simulink model "Fluxo_de_massa"  (R2025b)
settings: Solver=VariableStepAuto  StartTime=0.0  StopTime=10.0  RelTol=1e-3
undefined symbols (not defined in the file): N, Vd
settings Model: Creator=ivomu  LastModifiedBy=ivomu

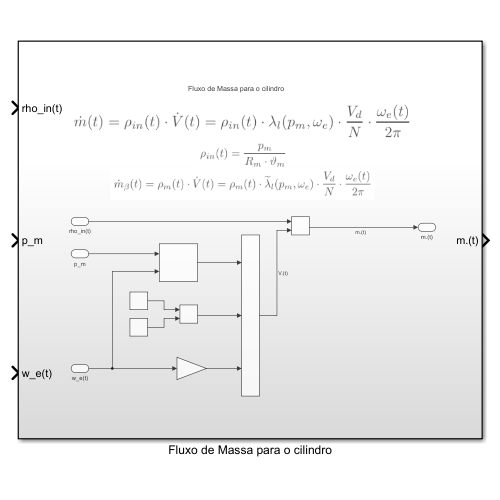
[thumbnail: Simulink's stored preview of the top-level diagram]
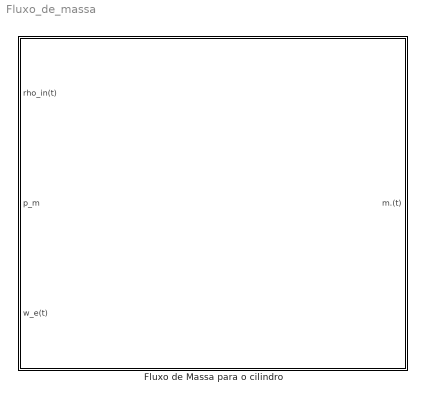
== system Fluxo_de_massa ==
  Fluxo de Massa para o cilindro : Subsystem

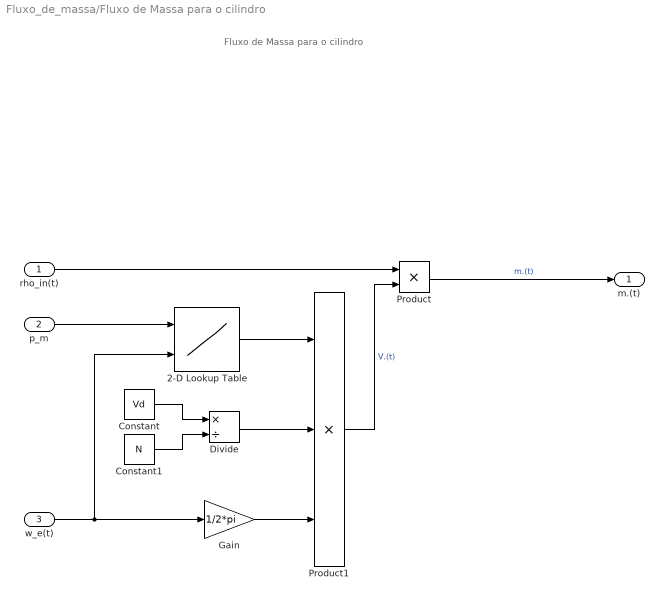
== system Fluxo_de_massa/Fluxo de Massa para o cilindro ==
  note: Fluxo de Massa para o cilindro
  rho_in(t) : Inport
  p_m : Inport  Port=2
  w_e(t) : Inport  Port=3
  2-D Lookup Table : Lookup_n-D  BreakpointsForDimension1=[1:3]  BreakpointsForDimension2=[1:3]  InternalRulePriority=Speed  RndMeth=Simplest
      settings: InputPortMap=u0,u1
  Constant : Constant  Value=Vd
  Constant1 : Constant  Value=N
  Divide : Product  Inputs=*/
  Gain : Gain  Gain=1/2*pi
  Product : Product
  Product1 : Product  Inputs=3
  m.(t) : Outport
  wires:
  rho_in(t)/1 -> Product/1
  Product1/1 -> Product/2  "V.(t)"
  p_m/1 -> 2-D Lookup Table/1
  Constant1/1 -> Divide/2
  Constant/1 -> Divide/1
  Gain/1 -> Product1/3
  Divide/1 -> Product1/2
  2-D Lookup Table/1 -> Product1/1
  Product/1 -> m.(t)/1  "m.(t)"
  w_e(t)/1 -> 2-D Lookup Table/2, Gain/1
